simulink model "StanfordArmModel"  (R2019b)
settings: Solver=FixedStepAuto  StartTime=0.0  StopTime=inf  RelTol=1e-3
libraries: simulink x8
settings Model: PacingRate=0.890000  Creator=crbon  LastModifiedBy=Chris

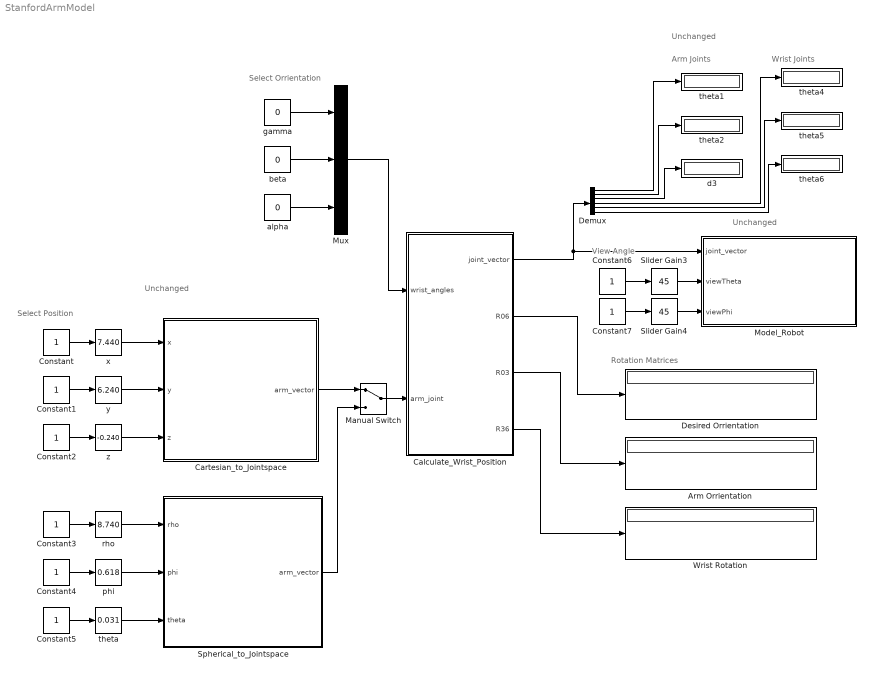
== system StanfordArmModel ==
  note: Unchanged
  note: Arm Joints
  note: Wrist Joints
  note: Rotation Matrices
  note: Select Orrientation
  note: Select Position
  note: View Angle
  note: Unchanged
  note: Unchanged
  Arm Orrientation : Display
  Calculate_Wrist_Position : MATLAB Function  TreatAsAtomicUnit=on
  Cartesian_to_Jointspace : MATLAB Function  TreatAsAtomicUnit=on
  Constant{,1..7} (8 alike) : Constant
  Demux : Demux  Outputs=6
  Desired Orrientation : Display
  Manual Switch : ManualSwitch
  Model_Robot : MATLAB Function  TreatAsAtomicUnit=on
  Mux : Mux  Inputs=3
  Slider Gain3 : simulink/Math Operations/Slider Gain  gain=45  low=-90  high=90
  Slider Gain4 : simulink/Math Operations/Slider Gain  gain=45  low=-90  high=90
  Spherical_to_Jointspace : MATLAB Function  TreatAsAtomicUnit=on
  Wrist Rotation : Display
  alpha : Constant  Value=0
  beta : Constant  Value=0
  d3 : Display
  gamma : Constant  Value=0
  phi : simulink/Math Operations/Slider Gain  gain=0.618  low=0  high=6.18
  "rho " : simulink/Math Operations/Slider Gain  gain=8.740  low=3  high=10
  theta : simulink/Math Operations/Slider Gain  gain=0.031  low=0  high=3.14
  theta{1..2,4..6} (5 alike) : Display
  x : simulink/Math Operations/Slider Gain  gain=7.440  low=-12  high=12
  y : simulink/Math Operations/Slider Gain  gain=6.240  low=-12  high=12
  z : simulink/Math Operations/Slider Gain  gain=-0.240  low=-12  high=12
  wires:
  Manual Switch/1 -> Calculate_Wrist_Position/2(arm_joint)
  Cartesian_to_Jointspace/1(arm_vector) -> Manual Switch/1
  Constant/1 -> x/1
  Constant1/1 -> y/1
  Constant2/1 -> z/1
  Constant5/1 -> theta/1
  Constant4/1 -> phi/1
  Constant3/1 -> "rho "/1
  x/1 -> Cartesian_to_Jointspace/1(x)
  y/1 -> Cartesian_to_Jointspace/2(y)
  z/1 -> Cartesian_to_Jointspace/3(z)
  "rho "/1 -> Spherical_to_Jointspace/1(rho)
  phi/1 -> Spherical_to_Jointspace/2(phi)
  theta/1 -> Spherical_to_Jointspace/3(theta)
  Spherical_to_Jointspace/1(arm_vector) -> Manual Switch/2
  Slider Gain4/1 -> Model_Robot/3(viewPhi)
  Slider Gain3/1 -> Model_Robot/2(viewTheta)
  Constant7/1 -> Slider Gain4/1
  Constant6/1 -> Slider Gain3/1
  alpha/1 -> Mux/3
  gamma/1 -> Mux/1
  beta/1 -> Mux/2
  Mux/1 -> Calculate_Wrist_Position/1(wrist_angles)
  Calculate_Wrist_Position/1(joint_vector) -> Model_Robot/1(joint_vector), Demux/1
  Demux/1 -> theta1/1
  Demux/2 -> theta2/1
  Demux/3 -> d3/1
  Demux/4 -> theta4/1
  Demux/5 -> theta5/1
  Demux/6 -> theta6/1
  Calculate_Wrist_Position/2(R06) -> Desired Orrientation/1
  Calculate_Wrist_Position/3(R03) -> Arm Orrientation/1
  Calculate_Wrist_Position/4(R36) -> Wrist Rotation/1

== matlab function StanfordArmModel/Cartesian_to_Jointspace ==
  data: x input; y input; z input; arm_vector output
% creates a joint vector for the position of the stanford arm from 
% a cartesian input; doesn't calculate wrist angles or EOAT
function arm_vector  = Cartesian_to_Jointspace(x,y,z)
%% initialize
arm_vector = zeros(1,3);

%% Calculate spherical
phi = atan2(y,x);
rho = sqrt(x.^2 + y.^2 + z.^2);
theta = acos(z/rho);

%% d3 
if (rho < 2)
    rho = 2;
end
d3 = sqrt(rho^2-4);
arm_vector(3) = d3;

%% theta2
theta_bound = pi/2-atan2(d3,2);
if (theta <= theta_bound)
    theta = theta_bound + 0.01;
elseif (theta >= pi-theta_bound)
    theta = pi-theta_bound - 0.01;
end
theta2 = acos(rho*cos(theta)/d3);
arm_vector(2) = theta2;

%% theta1
alpha = atan2(2,d3*sin(theta2));

theta1 = phi - alpha;
arm_vector(1) = theta1;
end

== matlab function StanfordArmModel/Model_Robot ==
  data: joint_vector input; viewTheta input; viewPhi input
function Model_Robot(joint_vector, viewTheta, viewPhi)

%% Unpack Joint Vector
theta1 = joint_vector(1);
theta2 = joint_vector(2);
d3     = joint_vector(3);
theta4 = joint_vector(4);
theta5 = joint_vector(5);
theta6 = joint_vector(6);

%% Calculate endpoints for visualization
% Cartesian
x = cos(theta1)*d3*sin(theta2)-sin(theta1)*2;
y = sin(theta1)*d3*sin(theta2)+cos(theta1)*2;
z = d3*cos(theta2);

% Spherical
Rho = sqrt(d3^2+4);
% Max elevation for current value of d3
phi_max = atan(d3/2);
% create surface spherical shell for current d3
Phi_grid=linspace(-phi_max,phi_max);
Theta_grid=linspace(0,2*pi);
[Phi_grid,Theta_grid]=meshgrid(Phi_grid,Theta_grid);
[X,Y,Z]=sph2cart(Theta_grid,Phi_grid,Rho);

% Polar unreachable zone
R = 2;
Z_grid = linspace(-15,15);
Theta_grid=linspace(0,2*pi);
[Theta_grid, Z_grid] = meshgrid(Theta_grid, Z_grid);
[Xp,Yp,Zp] = pol2cart(Theta_grid, R, Z_grid);

%% Define Links/ Robot Shapes
origin = [0;0;0];

Base  = [...
         -1  -1  -1  -1  -1   1   1  -1   1   1  -1   1   1  -1   1   1;...
          1  -1  -1   1   1   1   1   1   1  -1  -1  -1  -1  -1  -1   1;...
        -15 -15  -1  -1 -15 -15  -1  -1  -1  -1  -1  -1 -15 -15 -15 -15;...
];

Link1 = [...
          1  -1  -1   1   1   1   1   1   1  -1  -1  -1  -1  -1  -1   1;...
          1   1  -1  -1   1   1  -1  -1  -1  -1  -1  -1   1   1   1   1;...
         -1  -1  -1  -1  -1   1   1  -1   1   1  -1   1   1  -1   1   1;...
];

% Link1 = [...
%          .5 -.5 -.5  .5  .5  .5  .5  .5  .5 -.5 -.5 -.5 -.5 -.5 -.5  .5;...
%           2   2   1   1   2   2   1   1   1   1   1   1   2   2   2   2;...
%         -.5 -.5 -.5 -.5 -.5  .5  .5 -.5  .5  .5 -.5  .5  .5 -.5  .5  .5;...
% ];

Link2 = [...
          1  -1  -1   1   1   1   1   1   1  -1  -1  -1  -1  -1  -1   1;...
          1   1  -1  -1   1   1  -1  -1  -1  -1  -1  -1   1   1   1   1;...
         -1  -1  -1  -1  -1   1   1  -1   1   1  -1   1   1  -1   1   1;...
];

%no visible link in model
Link3 = [0;0;0];

Link4 = [...
        -.5 -.5 -.5 -.5 -.5  .5  .5 -.5  .5  .5 -.5  .5  .5 -.5  .5  .5;...
         .5 -.5 -.5  .5  .5  .5  .5  .5  .5 -.5 -.5 -.5 -.5 -.5 -.5  .5;...
        -15 -15  -1  -1 -15 -15  -1  -1  -1  -1  -1  -1 -15 -15 -15 -15;...
];

Link5 = [...
          1  -1  -1   1   1   1   1   1   1  -1  -1  -1  -1  -1  -1   1;...
          1   1  -1  -1   1   1  -1  -1  -1  -1  -1  -1   1   1   1   1;...
         -1  -1  -1  -1  -1   1   1  -1   1   1  -1   1   1  -1   1   1;...
];

Link6 = [...
        -.5 -.5 -.5 -.5 -.5  .5  .5 -.5  .5  .5 -.5  .5  .5 -.5  .5  .5;...
         .5 -.5 -.5  .5  .5  .5  .5  .5  .5 -.5 -.5 -.5 -.5 -.5 -.5  .5;...
          4   4   1   1   4   4   1   1   1   1   1   1   4   4   4   4;...
];

% shape of axis figure for base and EOAT
axes  = [...
         0 1.5 0  0  0  0  0;...
         0  0  0 1.5 0  0  0;...
         0  0  0  0  0 1.5 0;...
];

%% Transform Link 1
BaseLink1= TRANS01SF(Link1 ,theta1);

%% Transform Link 2
Link12   = TRANS12SF(Link2 ,theta2);
BaseLink2= TRANS01SF(Link12,theta1);
BaseLink2O = TRANS01SF(TRANS12SF(origin,theta2),theta1);

%% Transform Link 3
%no visible links
%   Link23   = TRANS23SF(Link3 ,d3    );
%   Link13   = TRANS12SF(Link23,theta2);
%   BaseLink3= TRANS01SF(Link13,theta1);
BaseLink3O = TRANS01SF(TRANS12SF(TRANS23SF(origin,d3),theta2),theta1);

%% Transform Link 4
Link34   = TRANS34SF(Link4 ,theta4);
Link24   = TRANS23SF(Link34,d3    );
Link14   = TRANS12SF(Link24,theta2);
BaseLink4= TRANS01SF(Link14,theta1);

%% Transform Link 5
Link45   = TRANS45SF(Link5 ,theta5);
Link35   = TRANS34SF(Link45,theta4);
Link25   = TRANS23SF(Link35,d3    );
Link15   = TRANS12SF(Link25,theta2);
BaseLink5= TRANS01SF(Link15,theta1);

%% Transform Link 6
Link56   = TRANS56SF(Link6 ,theta6);
Link46   = TRANS45SF(Link56,theta5);
Link36   = TRANS34SF(Link46,theta4);
Link26   = TRANS23SF(Link36,d3    );
Link16   = TRANS12SF(Link26,theta2);
BaseLink6= TRANS01SF(Link16,theta1);

%% Transform EOAT
Link67   = TRANS67SF(axes         );
Link57   = TRANS56SF(Link67,theta6);
Link47   = TRANS45SF(Link57,theta5);
Link37   = TRANS34SF(Link47,theta4);
Link27   = TRANS23SF(Link37,d3    );
Link17   = TRANS12SF(Link27,theta2);
BaseEOAT = TRANS01SF(Link17,theta1);


%% Plotting
plot3(Base(1,:),Base(2,:),Base(3,:),'k-')
axis([-15 15 -15 15 -15 15]);
grid on
hold on
plot3(BaseLink1(1,:),BaseLink1(2,:),BaseLink1(3,:),'b-', 'LineWidth', 2)
plot3(BaseLink2(1,:),BaseLink2(2,:),BaseLink2(3,:),'g-', 'LineWidth', 2)
%   plot3(BaseLink3(1,:),BaseLink3(2,:),BaseLink3(3,:),'k-', 'LineWidth', 2)
plot3(BaseLink4(1,:),BaseLink4(2,:),BaseLink4(3,:),'m-', 'LineWidth', 2)
plot3(BaseLink5(1,:),BaseLink5(2,:),BaseLink5(3,:),'b-', 'LineWidth', 2)
plot3(BaseLink6(1,:),BaseLink6(2,:),BaseLink6(3,:),'k-', 'LineWidth', 2)
plot3(BaseLink2O(1,:),BaseLink2O(2,:),BaseLink2O(3,:),'r*', 'LineWidth', 2)
plot3(BaseLink3O(1,:),BaseLink3O(2,:),BaseLink3O(3,:),'r*', 'LineWidth', 2)
plot3(axes(1,:),   axes(2,:),   axes(3,:),   'r-', 'LineWidth', 2)
plot3(axes(1,1),   axes(2,1),   axes(3,1),   'r*', 'LineWidth', 2)
plot3(BaseEOAT(1,:), BaseEOAT(2,:), BaseEOAT(3,:), 'r-', 'LineWidth', 2)
plot3(BaseEOAT(1,1), BaseEOAT(2,1), BaseEOAT(3,1), 'r*', 'LineWidth', 2)
surf(X,Y,Z, 'EdgeColor', 'none');
alpha 0.1
surf(Xp,Yp,Zp, 'EdgeColor', 'none');
alpha 0.2
% draws line to wrist
% plot3([0 x],[0 y],[0 z],'k-', 'LineWidth',4)
xlabel('X');
ylabel('Y');
zlabel('Z');
view(viewTheta,viewPhi);
hold off

end

== matlab function StanfordArmModel/Spherical_to_Jointspace ==
  data: rho input; phi input; theta input; arm_vector output
% creates a joint vector for the position of the stanford arm from 
% a spherical input; doesn't calculate wrist angles or EOAT
function arm_vector  = Spherical_to_Jointspace(rho,phi,theta)
%% initialize
arm_vector = zeros(1,3);

%% d3
if (rho < 2)
    rho = 2;
end
d3 = sqrt(rho^2-4);
arm_vector(3) = d3;

%% theta2
theta_bound = pi/2-atan2(d3,2);
if (theta <= theta_bound)
    theta = theta_bound + 0.01;
elseif (theta >= pi-theta_bound)
    theta = pi-theta_bound - 0.01;
end
theta2 = acos(rho*cos(theta)/d3);
arm_vector(2) = theta2;

%% theta1
alpha = atan2(2,d3*sin(theta2));

theta1 = phi - alpha;
arm_vector(1) = theta1;
end

== matlab function StanfordArmModel/Calculate_Wrist_Position ==
  data: wrist_angles input; arm_joint input; joint_vector output; R06 output; R03 output; R36 output
function [joint_vector,R06,R03,R36]  = Calculate_Wrist_Position(wrist_angles, arm_joint)

%%Initialize Joint Vector
joint_vector = zeros(1,6);

%% Unpack Joint Vector
theta1 = arm_joint(1);
theta2 = arm_joint(2);
d3     = arm_joint(3);

%% Unpack Desired Wrist Vector
Gamma  = wrist_angles(1);
Beta   = wrist_angles(2);
Alpha  = wrist_angles(3);

%% Find R03
R03 = R03SF(theta1,theta2);
R03 = round(R03*1000)/1000;

%% Calculate Desired orrientation
R06 = R36SF(Gamma,Beta,Alpha);
R06 = round(R06*1000)/1000;

%% Get R36
R36 = R03'*R06;
r = round(R36*1000)/1000;

%% Calculate theta4, theta5, theta6
theta5 = atan2(sqrt(r(3,1)^2+r(3,2)^2),r(3,3));
theta5 = round(theta5*1000)/1000;
if (theta5 ~= 0)
    theta4 = atan2(r(2,3)/sin(theta5), r(1,3)/sin(theta5));
    theta6 = atan2(r(3,2)/sin(theta5),-r(3,1)/sin(theta5));
else
   theta4 = 0;
   theta6 = atan2(-r(1,2),r(1,1));
end
    
%% Make Joint Vector
joint_vector(1:3) = arm_joint;
joint_vector(4:6) = [theta4,theta5,theta6];

end
